simulink model "vehicle_sim"  (R2023a)
settings: Solver=VariableStepAuto  StartTime=0.0  StopTime=1.4  RelTol=1e-3
values from neighbouring files (symbols this model uses):
  th = [m;d;a;b;Izz;h;Ixz;dr;df;rw;kt;kb;Cf;Cr;chi;sigma;g]    [vehicle_sim_main.m]
  u_delta_step = 10*pi/180    (= 0.174532925199)    [vehicle_sim_main.m]
  z0 = [w;mu;vx;vy;r;delta;psi]    [vehicle_sim_main.m]
settings Model: Creator=Lorenzo  LastModifiedBy=andre
settings SolverCC: AlgebraicLoopSolver=TrustRegion
settings DataIOCC: ReturnWorkspaceOutputs=off
settings DebuggingCC: UnconnectedInputMsg=warning  UnconnectedOutputMsg=warning  UnconnectedLineMsg=warning  ArithmeticOperatorsInVariantConditions=warning
settings ModelReferenceCC: EnableRefExpFcnMdlSchedulingChecks=on
settings SFSimCC: CustomCodeUndefinedFunction=UseInterfaceOnly

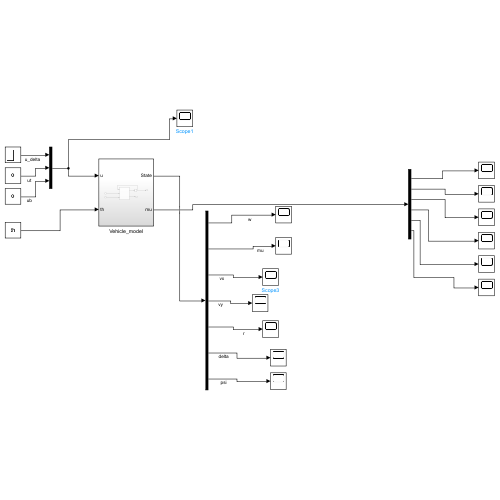
[thumbnail: Simulink's stored preview of the top-level diagram]
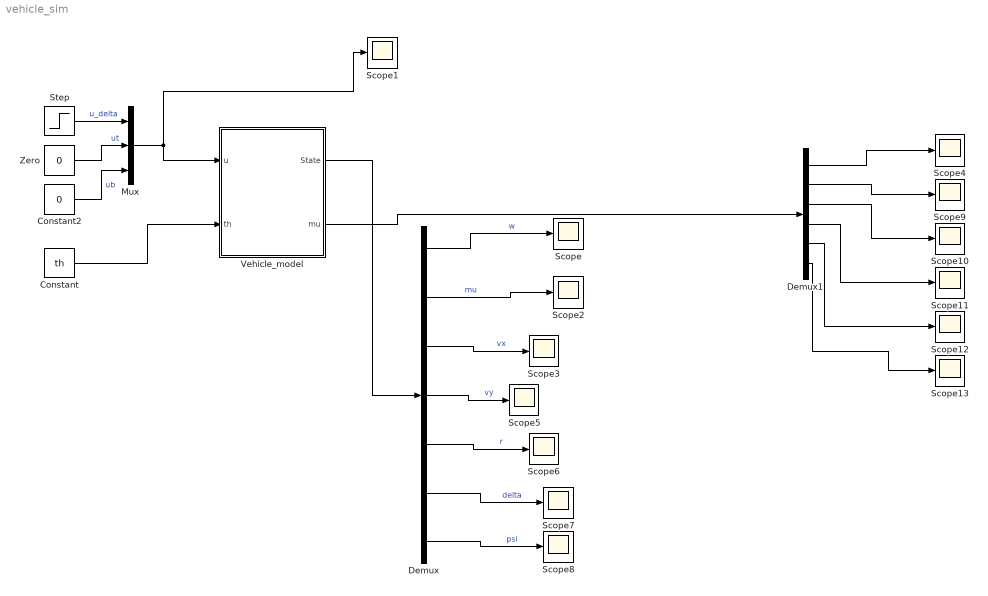
== system vehicle_sim ==
  Constant : Constant  Value=th
  Constant2 : Constant  Value=0
  Demux : Demux  Outputs=7
  Demux1 : Demux  Outputs=6
  Mux : Mux  Inputs=3
  Scope{,1..13} (14 alike) : Scope
  Step : Step  Time=0  After=u_delta_step/10  SampleTime=0
  Vehicle_model : Subsystem
  Zero : Constant  Value=0  OutDataTypeStr=Inherit: Inherit via back propagation
  wires:
  Vehicle_model/1(State) -> Demux/1
  Step/1 -> Mux/1  "u_delta"
  Zero/1 -> Mux/2  "ut"
  Constant2/1 -> Mux/3  "ub"
  Constant/1 -> Vehicle_model/2(th)
  Mux/1 -> Vehicle_model/1(u), Scope1/1
  Demux/1 -> Scope/1  "w"
  Demux/2 -> Scope2/1  "mu"
  Demux/3 -> Scope3/1  "vx"
  Demux/7 -> Scope8/1  "psi"
  Demux/6 -> Scope7/1  "delta"
  Demux/5 -> Scope6/1  "r"
  Demux/4 -> Scope5/1  "vy"
  Vehicle_model/2(mu) -> Demux1/1
  Demux1/1 -> Scope4/1
  Demux1/2 -> Scope9/1
  Demux1/3 -> Scope10/1
  Demux1/4 -> Scope11/1
  Demux1/5 -> Scope12/1
  Demux1/6 -> Scope13/1

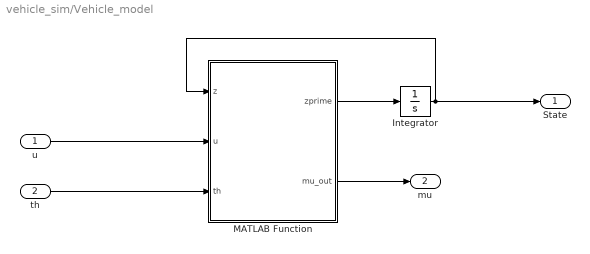
== system vehicle_sim/Vehicle_model ==
  u : Inport
  th : Inport  Port=2
  Integrator : Integrator  InitialCondition=z0
  MATLAB Function : MATLAB Function  TreatAsAtomicUnit=on
  State : Outport  VectorParamsAs1DForOutWhenUnconnected=off
  mu : Outport  Port=2
  wires:
  Integrator/1 -> MATLAB Function/1(z), State/1
  MATLAB Function/1(zprime) -> Integrator/1
  u/1 -> MATLAB Function/2(u)
  th/1 -> MATLAB Function/3(th)
  MATLAB Function/2(mu_out) -> mu/1

== matlab function vehicle_sim/Vehicle_model/MATLAB Function ==
  data: z input; u input; zprime output; th input; mu_out output
function [zprime,mu_out] =vehicle_dynamics(z,u,th)        %For the time being, assume no disturbances
% Nonlinear dynamic model of a road vehicle with six states: 
% w: is the distance of the com to the center line 
% mu: is the local heading angle 
% vx: is the longitudinal velocity of the com 
% vy: is the lateral velocity of the com 
% r: is the yaw rate
% Delta: is the steering angle 
% Model for lateral and longitudinal tire forces is in another function 

% Inputs:
%           z      (model state)
%           u       (steering rate u_delta, braking coefficient torque ub, traction coefficient torque ut),         
%           th      (model parameters)
%
% Outputs:  z_dot  (derivative of the state with respect to time)
%           F       (longitudinal and lateral forces)

%% Read parameters, states and inputs
% Parameters      
m       =       th(1,1);     % vehicle mass (kg)
d       =       th(2,1);     % distance along yb from the com and the longitudinal axle (m)
a       =       th(3,1);     % distance between center of gravity and front axle (m)
b       =       th(4,1);     % distance between center of gravity and rear axle (m)
Izz     =       th(5,1);     % vehicle moment of inertia with respect to z-axis (kg*m^2)
h       =       th(6,1);     % height of the com from the ground (m)
Ixz     =       th(7,1);     % vehicle moment of inertia with respect to x-z plane (kg*m^2)
dr      =       th(8,1);     % half of the rear truck width (m)
df      =       th(9,1);     % half of the front truck width (m)
rw      =       th(10,1);    % wheel radius (m)
kt      =       th(11,1);    % traction ratio - typically 0
kb      =       th(12,1);    % brake ratio - typically 0.5
Cf      =       th(13,1);    % pseudo-cornering stiffness of the front wheel 
Cr      =       th(14,1);    % pseudo-cornering stiffness of the rear wheel
chi     =       th(15,1);    % local center line angle
sigma   =       th(16,1);    % curvature (m^-1)
g       =       th(17,1);    % gravity acceleration (m/s^2)

l       =       a+b;         % wheelbase (m)
Izz_tilde=      Izz+m*(b^2+d^2);
Ixz_tilde=      Ixz+m*b*h;


% States

w       =       z(1,1);    % displacement transverse to the center line (m)
mu      =       z(2,1);    % local heading angle (rad) 
vx      =       z(3,1);    % inertial X velocity (m/s)
vy      =       z(4,1);    % inertial Y velocity (m/s)
r       =       z(5,1);    % yaw rate (rad/s)
delta   =       z(6,1);    % steering angle (rad)
psi     =       z(7,1);    % yaw angle(rad)      

% Inputs
u_delta      =       u(1,1);     % steering yaw rate (rad/s)
ub           =       u(2,1);     % braking coefficient torque 
ut           =       u(3,1);     % traction coeffient torque

%% Compute friction coefficients
beta        =   atan2(vy,vx);           % com side-slip angle (rad)
v           =   sqrt(vx^2+vy^2);        % com velocity (m/s)

beta_rr     =   beta+(rw*b)/v;          % rear-right wheel side-slip angle (rad)
beta_rl     =   beta_rr;                % rear-left wheel side-slip angle (rad)
beta_fr     =   beta+delta-(rw*a)/v;    % front-right wheel-slip angle  (rad)
beta_fl     =   beta_fr;                % front-left wheel-slip angle (rad)

%longitudinal friction coefficients
mux_fl       =   kt*ut-kb*ub;            % longitudinal friction coefficient of the front-left wheel
mux_fr       =   mux_fl;                 % longitudinal friction coefficient of the front-right wheel
mux_rl       =   (1-kt)*ut-(1-kb)*ub;    % longitudinal friction coefficient of the front-left wheel
mux_rr       =   mux_rl;                 % longitudinal friction coefficient of the front-right wheel

%lateral friction coefficients
muy_fl       =  Cf*beta_fl;             % lateral friction coefficient of the front-left wheel    
muy_fr       =  Cf*beta_fr;             % lateral friction coefficient of the front-right wheel
muy_rl       =  Cr*beta_rl;             % lateral friction coefficient of the rear-left wheel    
muy_rr       =  Cr*beta_rr;             % lateral friction coefficient of the rear-right wheel

%Equivalent friction coefficients that come from the dynamic equation
mu_tilde_x_fl       =  mux_fl*cos(delta)-muy_fl*sin(delta);            % equivalent longitudinal friction coefficient of the front-left wheel
mu_tilde_x_fr       =  mux_fr*cos(delta)-muy_fr*sin(delta);            % equivalent longitudinal friction coefficient of the front-right wheel
mu_tilde_y_fl       =  mux_fl*sin(delta)+muy_fl*cos(delta);                          % equivalent lateral friction coefficient of the front-left wheel
mu_tilde_y_fr       =  mux_fr*sin(delta)+muy_fr*cos(delta);                                       % equivalent lateral friction coefficient of the front-right wheel

muxy_fr      =  l*muy_fr - df*mux_fr;
muxy_fl      =  l*muy_fl + df*mux_fl;

%% Matrix for the dynamic equations
%I will write the matrices for the linear equation Ax=B, so that x=A^-1*B

A           = zeros(8,8);
A(1,:)      = [m, 0, -m*d, 0, mu_tilde_x_fr, mu_tilde_x_fl, mux_rr, mux_rl];
A(2,:)      = [0, m, m*b, 0,  mu_tilde_y_fr, mu_tilde_y_fl, muy_rr, muy_rl];
A(3,:)      = [-m*d, m*b, Izz_tilde, 0, muxy_fr, muxy_fl, -dr*mux_rr, dr*mux_rl];
A(4,4)      = 1;
A(5,:)      = [0, 0, 0, 0, -1, -1, -1, -1];
A(6,:)      = [0, m*h, Ixz_tilde, 0, -df, df, -dr, dr];
A(7,:)      = [-m*h, 0, m*h*d, 0, l, l, 0, 0];
A(8,:)      = [0, 0, 0, 0, -dr, dr, df, -df];

% A           = zeros(8,8);
% A(1,:)      = [m, 0, -m*d, 0, 1, 1.1, 1.12, 1.2];
% A(2,:)      = [0, m, m*b, 0,  1.1, 1.2, 1.21, 1.14];
% A(3,:)      = [-m*d, m*b, Izz_tilde, 0, 1.2, 1.19, -dr*1.12, dr*1.21];
% A(4,4)      = 1;
% A(5,:)      = [0, 0, 0, 0, -1, -1, -1, -1];
% A(6,:)      = [0, m*h, Ixz_tilde, 0, -df, df, -dr, dr];
% A(7,:)      = [-m*h, 0, m*h*d, 0, l, l, 0, 0];
% A(8,:)      = [0, 0, 0, 0, -dr, dr, df, -df];

B           = zeros(8,1);
B(1,1)      = m*r*(vy+b*r);
B(2,1)      = -m*r*(vx-d*r);
B(3,1)      = -m*r*(d*vy+b*vx);
B(4,1)      = u_delta;
B(5,1)      = m*g;
B(6,1)      = m*g*d-m*h*r*(vx-d*r);
B(7,1)      = -m*g*b-m*h*vy*r-Ixz_tilde*r^2;

unk         = (A^-1)*B;                                                       % unk stands for "unknown"

zdot=zeros(7,1);
zdot(1,1)   = vx*sin(psi-chi)+vy*cos(psi-chi);                              % w_dot (m/s) - time derivative of the displacement transverse to the center line (aka transversal speed)
zdot(2,1)   = r - sigma*(vx*cos(psi-chi)-vy*sin(psi-chi))/(1-sigma*w);      % mu_dot (rad/s) - time derivative of the heading angle
zdot(3,1)   = unk(3,1);                                                     % vx_dot (m/s) - longitudinal velocity 
zdot(4,1)   = unk(4,1);                                                     % vy_dot (m/s) - lateral velocity
zdot(5,1)   = unk(5,1);                                                     % r_dot (rad/s) - yaw acceleration
zdot(6,1)   = unk(6,1);                                                     % delta_dot(rad/s) - steering rate 
zdot(7,1)   = r;                                                            % r (rad/s) - yaw rate

s_dot_inv   =   (1-sigma*w)/(vx*cos(psi-chi)-vy*sin(psi-chi));
zprime = zdot * s_dot_inv;

%% Temporary part

mu_out=[mu_tilde_x_fl; mu_tilde_x_fr; mu_tilde_y_fl; mu_tilde_y_fr; muxy_fr; muxy_fl];
